simulink model "c00004M_harness"  (R2018a)
settings: Solver=FixedStepAuto  StartTime=0.0  StopTime=300  FixedStep=0.1  RelTol=1e-3
undefined symbols (not defined in the file): A1, hmax, R1, R2, sigbuilder_block, TempThreshold
(part 4 of 14)

== system c00004M_harness/M176/Tank3 ==
  CT3 : Inport
  F3 : Inport  Port=2
  E3 : Inport  Port=3
  MR3 : Inport  Port=4
  T3 : Inport  Port=5
  EB3 : Inport  Port=6
  Control : Subsystem
  Memory : Memory
  TankModel : Subsystem
  LL3 : Outport
  wires:
  TankModel/1(LiquidLevel) -> Memory/1, LL3/1
  Control/2(LiquidOut) -> TankModel/2(LiquidOut)
  Memory/1 -> Control/8(LiquidLevel)
  MR3/1 -> Control/3(ManualReference)
  CT3/1 -> Control/2(StartMaintenance), Control/1(ControlType)
  F3/1 -> Control/4(Fill)
  E3/1 -> Control/5(Empty)
  EB3/1 -> Control/6(EmergencyButton)
  T3/1 -> Control/7(Temperature)
  Control/1(LiquidIn) -> TankModel/1(LiquidIn)

== system c00004M_harness/M177/Tank3 ==
  CT3 : Inport
  F3 : Inport  Port=2
  E3 : Inport  Port=3
  MR3 : Inport  Port=4
  T3 : Inport  Port=5
  EB3 : Inport  Port=6
  Control : Subsystem
  Memory : Memory
  TankModel : Subsystem
  LL3 : Outport
  wires:
  TankModel/1(LiquidLevel) -> Memory/1, LL3/1
  Control/2(LiquidOut) -> TankModel/2(LiquidOut)
  Memory/1 -> Control/8(LiquidLevel)
  MR3/1 -> Control/3(ManualReference)
  CT3/1 -> Control/2(StartMaintenance), Control/1(ControlType)
  F3/1 -> Control/4(Fill)
  E3/1 -> Control/5(Empty)
  EB3/1 -> Control/6(EmergencyButton)
  T3/1 -> Control/7(Temperature)
  Control/1(LiquidIn) -> TankModel/1(LiquidIn)

== system c00004M_harness/M178/Tank3 ==
  CT3 : Inport
  F3 : Inport  Port=2
  E3 : Inport  Port=3
  MR3 : Inport  Port=4
  T3 : Inport  Port=5
  EB3 : Inport  Port=6
  Control : Subsystem
  Memory : Memory
  TankModel : Subsystem
  LL3 : Outport
  wires:
  TankModel/1(LiquidLevel) -> Memory/1, LL3/1
  Control/2(LiquidOut) -> TankModel/2(LiquidOut)
  Memory/1 -> Control/8(LiquidLevel)
  MR3/1 -> Control/3(ManualReference)
  CT3/1 -> Control/2(StartMaintenance), Control/1(ControlType)
  F3/1 -> Control/4(Fill)
  E3/1 -> Control/5(Empty)
  EB3/1 -> Control/6(EmergencyButton)
  T3/1 -> Control/7(Temperature)
  Control/1(LiquidIn) -> TankModel/1(LiquidIn)

== system c00004M_harness/M179/Tank3 ==
  CT3 : Inport
  F3 : Inport  Port=2
  E3 : Inport  Port=3
  MR3 : Inport  Port=4
  T3 : Inport  Port=5
  EB3 : Inport  Port=6
  Control : Subsystem
  Memory : Memory
  TankModel : Subsystem
  LL3 : Outport
  wires:
  TankModel/1(LiquidLevel) -> Memory/1, LL3/1
  Control/2(LiquidOut) -> TankModel/2(LiquidOut)
  Memory/1 -> Control/8(LiquidLevel)
  MR3/1 -> Control/3(ManualReference)
  CT3/1 -> Control/2(StartMaintenance), Control/1(ControlType)
  F3/1 -> Control/4(Fill)
  E3/1 -> Control/5(Empty)
  EB3/1 -> Control/6(EmergencyButton)
  T3/1 -> Control/7(Temperature)
  Control/1(LiquidIn) -> TankModel/1(LiquidIn)

== system c00004M_harness/M180/Tank3 ==
  CT3 : Inport
  F3 : Inport  Port=2
  E3 : Inport  Port=3
  MR3 : Inport  Port=4
  T3 : Inport  Port=5
  EB3 : Inport  Port=6
  Control : Subsystem
  Memory : Memory
  TankModel : Subsystem
  LL3 : Outport
  wires:
  TankModel/1(LiquidLevel) -> Memory/1, LL3/1
  Control/2(LiquidOut) -> TankModel/2(LiquidOut)
  Memory/1 -> Control/8(LiquidLevel)
  MR3/1 -> Control/3(ManualReference)
  CT3/1 -> Control/2(StartMaintenance), Control/1(ControlType)
  F3/1 -> Control/4(Fill)
  E3/1 -> Control/5(Empty)
  EB3/1 -> Control/6(EmergencyButton)
  T3/1 -> Control/7(Temperature)
  Control/1(LiquidIn) -> TankModel/1(LiquidIn)

== system c00004M_harness/M181/Tank3 ==
  CT3 : Inport
  F3 : Inport  Port=2
  E3 : Inport  Port=3
  MR3 : Inport  Port=4
  T3 : Inport  Port=5
  EB3 : Inport  Port=6
  Control : Subsystem
  Memory : Memory
  TankModel : Subsystem
  LL3 : Outport
  wires:
  TankModel/1(LiquidLevel) -> Memory/1, LL3/1
  Control/2(LiquidOut) -> TankModel/2(LiquidOut)
  Memory/1 -> Control/8(LiquidLevel)
  MR3/1 -> Control/3(ManualReference)
  CT3/1 -> Control/2(StartMaintenance), Control/1(ControlType)
  F3/1 -> Control/4(Fill)
  E3/1 -> Control/5(Empty)
  EB3/1 -> Control/6(EmergencyButton)
  T3/1 -> Control/7(Temperature)
  Control/1(LiquidIn) -> TankModel/1(LiquidIn)

== system c00004M_harness/M182/Tank3 ==
  CT3 : Inport
  F3 : Inport  Port=2
  E3 : Inport  Port=3
  MR3 : Inport  Port=4
  T3 : Inport  Port=5
  EB3 : Inport  Port=6
  Control : Subsystem
  Memory : Memory
  TankModel : Subsystem
  LL3 : Outport
  wires:
  TankModel/1(LiquidLevel) -> Memory/1, LL3/1
  Control/2(LiquidOut) -> TankModel/2(LiquidOut)
  Memory/1 -> Control/8(LiquidLevel)
  MR3/1 -> Control/3(ManualReference)
  CT3/1 -> Control/2(StartMaintenance), Control/1(ControlType)
  F3/1 -> Control/4(Fill)
  E3/1 -> Control/5(Empty)
  EB3/1 -> Control/6(EmergencyButton)
  T3/1 -> Control/7(Temperature)
  Control/1(LiquidIn) -> TankModel/1(LiquidIn)

== system c00004M_harness/M183/Tank3 ==
  CT3 : Inport
  F3 : Inport  Port=2
  E3 : Inport  Port=3
  MR3 : Inport  Port=4
  T3 : Inport  Port=5
  EB3 : Inport  Port=6
  Control : Subsystem
  Memory : Memory
  TankModel : Subsystem
  LL3 : Outport
  wires:
  TankModel/1(LiquidLevel) -> Memory/1, LL3/1
  Control/2(LiquidOut) -> TankModel/2(LiquidOut)
  Memory/1 -> Control/8(LiquidLevel)
  MR3/1 -> Control/3(ManualReference)
  CT3/1 -> Control/2(StartMaintenance), Control/1(ControlType)
  F3/1 -> Control/4(Fill)
  E3/1 -> Control/5(Empty)
  EB3/1 -> Control/6(EmergencyButton)
  T3/1 -> Control/7(Temperature)
  Control/1(LiquidIn) -> TankModel/1(LiquidIn)

== system c00004M_harness/M184/Tank3 ==
  CT3 : Inport
  F3 : Inport  Port=2
  E3 : Inport  Port=3
  MR3 : Inport  Port=4
  T3 : Inport  Port=5
  EB3 : Inport  Port=6
  Control : Subsystem
  Memory : Memory
  TankModel : Subsystem
  LL3 : Outport
  wires:
  TankModel/1(LiquidLevel) -> Memory/1, LL3/1
  Control/2(LiquidOut) -> TankModel/2(LiquidOut)
  Memory/1 -> Control/8(LiquidLevel)
  MR3/1 -> Control/3(ManualReference)
  CT3/1 -> Control/2(StartMaintenance), Control/1(ControlType)
  F3/1 -> Control/4(Fill)
  E3/1 -> Control/5(Empty)
  EB3/1 -> Control/6(EmergencyButton)
  T3/1 -> Control/7(Temperature)
  Control/1(LiquidIn) -> TankModel/1(LiquidIn)

== system c00004M_harness/M185/Tank3 ==
  CT3 : Inport
  F3 : Inport  Port=2
  E3 : Inport  Port=3
  MR3 : Inport  Port=4
  T3 : Inport  Port=5
  EB3 : Inport  Port=6
  Control : Subsystem
  Memory : Memory
  TankModel : Subsystem
  LL3 : Outport
  wires:
  TankModel/1(LiquidLevel) -> Memory/1, LL3/1
  Control/2(LiquidOut) -> TankModel/2(LiquidOut)
  Memory/1 -> Control/8(LiquidLevel)
  MR3/1 -> Control/3(ManualReference)
  CT3/1 -> Control/2(StartMaintenance), Control/1(ControlType)
  F3/1 -> Control/4(Fill)
  E3/1 -> Control/5(Empty)
  EB3/1 -> Control/6(EmergencyButton)
  T3/1 -> Control/7(Temperature)
  Control/1(LiquidIn) -> TankModel/1(LiquidIn)

== system c00004M_harness/M186/Tank3 ==
  CT3 : Inport
  F3 : Inport  Port=2
  E3 : Inport  Port=3
  MR3 : Inport  Port=4
  T3 : Inport  Port=5
  EB3 : Inport  Port=6
  Control : Subsystem
  Memory : Memory
  TankModel : Subsystem
  LL3 : Outport
  wires:
  TankModel/1(LiquidLevel) -> Memory/1, LL3/1
  Control/2(LiquidOut) -> TankModel/2(LiquidOut)
  Memory/1 -> Control/8(LiquidLevel)
  MR3/1 -> Control/3(ManualReference)
  CT3/1 -> Control/2(StartMaintenance), Control/1(ControlType)
  F3/1 -> Control/4(Fill)
  E3/1 -> Control/5(Empty)
  EB3/1 -> Control/6(EmergencyButton)
  T3/1 -> Control/7(Temperature)
  Control/1(LiquidIn) -> TankModel/1(LiquidIn)

== system c00004M_harness/M187/Tank3 ==
  CT3 : Inport
  F3 : Inport  Port=2
  E3 : Inport  Port=3
  MR3 : Inport  Port=4
  T3 : Inport  Port=5
  EB3 : Inport  Port=6
  Control : Subsystem
  Memory : Memory
  TankModel : Subsystem
  LL3 : Outport
  wires:
  TankModel/1(LiquidLevel) -> Memory/1, LL3/1
  Control/2(LiquidOut) -> TankModel/2(LiquidOut)
  Memory/1 -> Control/8(LiquidLevel)
  MR3/1 -> Control/3(ManualReference)
  CT3/1 -> Control/2(StartMaintenance), Control/1(ControlType)
  F3/1 -> Control/4(Fill)
  E3/1 -> Control/5(Empty)
  EB3/1 -> Control/6(EmergencyButton)
  T3/1 -> Control/7(Temperature)
  Control/1(LiquidIn) -> TankModel/1(LiquidIn)

== system c00004M_harness/M188/Tank3 ==
  CT3 : Inport
  F3 : Inport  Port=2
  E3 : Inport  Port=3
  MR3 : Inport  Port=4
  T3 : Inport  Port=5
  EB3 : Inport  Port=6
  Control : Subsystem
  Memory : Memory
  TankModel : Subsystem
  LL3 : Outport
  wires:
  TankModel/1(LiquidLevel) -> Memory/1, LL3/1
  Control/2(LiquidOut) -> TankModel/2(LiquidOut)
  Memory/1 -> Control/8(LiquidLevel)
  MR3/1 -> Control/3(ManualReference)
  CT3/1 -> Control/2(StartMaintenance), Control/1(ControlType)
  F3/1 -> Control/4(Fill)
  E3/1 -> Control/5(Empty)
  EB3/1 -> Control/6(EmergencyButton)
  T3/1 -> Control/7(Temperature)
  Control/1(LiquidIn) -> TankModel/1(LiquidIn)

== system c00004M_harness/M189/Tank3 ==
  CT3 : Inport
  F3 : Inport  Port=2
  E3 : Inport  Port=3
  MR3 : Inport  Port=4
  T3 : Inport  Port=5
  EB3 : Inport  Port=6
  Control : Subsystem
  Memory : Memory
  TankModel : Subsystem
  LL3 : Outport
  wires:
  TankModel/1(LiquidLevel) -> Memory/1, LL3/1
  Control/2(LiquidOut) -> TankModel/2(LiquidOut)
  Memory/1 -> Control/8(LiquidLevel)
  MR3/1 -> Control/3(ManualReference)
  CT3/1 -> Control/2(StartMaintenance), Control/1(ControlType)
  F3/1 -> Control/4(Fill)
  E3/1 -> Control/5(Empty)
  EB3/1 -> Control/6(EmergencyButton)
  T3/1 -> Control/7(Temperature)
  Control/1(LiquidIn) -> TankModel/1(LiquidIn)

== system c00004M_harness/M190/Tank3 ==
  CT3 : Inport
  F3 : Inport  Port=2
  E3 : Inport  Port=3
  MR3 : Inport  Port=4
  T3 : Inport  Port=5
  EB3 : Inport  Port=6
  Control : Subsystem
  Memory : Memory
  TankModel : Subsystem
  LL3 : Outport
  wires:
  TankModel/1(LiquidLevel) -> Memory/1, LL3/1
  Control/2(LiquidOut) -> TankModel/2(LiquidOut)
  Memory/1 -> Control/8(LiquidLevel)
  MR3/1 -> Control/3(ManualReference)
  CT3/1 -> Control/2(StartMaintenance), Control/1(ControlType)
  F3/1 -> Control/4(Fill)
  E3/1 -> Control/5(Empty)
  EB3/1 -> Control/6(EmergencyButton)
  T3/1 -> Control/7(Temperature)
  Control/1(LiquidIn) -> TankModel/1(LiquidIn)

== system c00004M_harness/M191/Tank3 ==
  CT3 : Inport
  F3 : Inport  Port=2
  E3 : Inport  Port=3
  MR3 : Inport  Port=4
  T3 : Inport  Port=5
  EB3 : Inport  Port=6
  Control : Subsystem
  Memory : Memory
  TankModel : Subsystem
  LL3 : Outport
  wires:
  TankModel/1(LiquidLevel) -> Memory/1, LL3/1
  Control/2(LiquidOut) -> TankModel/2(LiquidOut)
  Memory/1 -> Control/8(LiquidLevel)
  MR3/1 -> Control/3(ManualReference)
  CT3/1 -> Control/2(StartMaintenance), Control/1(ControlType)
  F3/1 -> Control/4(Fill)
  E3/1 -> Control/5(Empty)
  EB3/1 -> Control/6(EmergencyButton)
  T3/1 -> Control/7(Temperature)
  Control/1(LiquidIn) -> TankModel/1(LiquidIn)

== system c00004M_harness/M192/Tank3 ==
  CT3 : Inport
  F3 : Inport  Port=2
  E3 : Inport  Port=3
  MR3 : Inport  Port=4
  T3 : Inport  Port=5
  EB3 : Inport  Port=6
  Control : Subsystem
  Memory : Memory
  TankModel : Subsystem
  LL3 : Outport
  wires:
  TankModel/1(LiquidLevel) -> Memory/1, LL3/1
  Control/2(LiquidOut) -> TankModel/2(LiquidOut)
  Memory/1 -> Control/8(LiquidLevel)
  MR3/1 -> Control/3(ManualReference)
  CT3/1 -> Control/2(StartMaintenance), Control/1(ControlType)
  F3/1 -> Control/4(Fill)
  E3/1 -> Control/5(Empty)
  EB3/1 -> Control/6(EmergencyButton)
  T3/1 -> Control/7(Temperature)
  Control/1(LiquidIn) -> TankModel/1(LiquidIn)

== system c00004M_harness/M193/Tank3 ==
  CT3 : Inport
  F3 : Inport  Port=2
  E3 : Inport  Port=3
  MR3 : Inport  Port=4
  T3 : Inport  Port=5
  EB3 : Inport  Port=6
  Control : Subsystem
  Memory : Memory
  TankModel : Subsystem
  LL3 : Outport
  wires:
  TankModel/1(LiquidLevel) -> Memory/1, LL3/1
  Control/2(LiquidOut) -> TankModel/2(LiquidOut)
  Memory/1 -> Control/8(LiquidLevel)
  MR3/1 -> Control/3(ManualReference)
  CT3/1 -> Control/2(StartMaintenance), Control/1(ControlType)
  F3/1 -> Control/4(Fill)
  E3/1 -> Control/5(Empty)
  EB3/1 -> Control/6(EmergencyButton)
  T3/1 -> Control/7(Temperature)
  Control/1(LiquidIn) -> TankModel/1(LiquidIn)

== system c00004M_harness/M194/Tank3 ==
  CT3 : Inport
  F3 : Inport  Port=2
  E3 : Inport  Port=3
  MR3 : Inport  Port=4
  T3 : Inport  Port=5
  EB3 : Inport  Port=6
  Control : Subsystem
  Memory : Memory
  TankModel : Subsystem
  LL3 : Outport
  wires:
  TankModel/1(LiquidLevel) -> Memory/1, LL3/1
  Control/2(LiquidOut) -> TankModel/2(LiquidOut)
  Memory/1 -> Control/8(LiquidLevel)
  MR3/1 -> Control/3(ManualReference)
  CT3/1 -> Control/2(StartMaintenance), Control/1(ControlType)
  F3/1 -> Control/4(Fill)
  E3/1 -> Control/5(Empty)
  EB3/1 -> Control/6(EmergencyButton)
  T3/1 -> Control/7(Temperature)
  Control/1(LiquidIn) -> TankModel/1(LiquidIn)

== system c00004M_harness/M195/Tank3 ==
  CT3 : Inport
  F3 : Inport  Port=2
  E3 : Inport  Port=3
  MR3 : Inport  Port=4
  T3 : Inport  Port=5
  EB3 : Inport  Port=6
  Control : Subsystem
  Memory : Memory
  TankModel : Subsystem
  LL3 : Outport
  wires:
  TankModel/1(LiquidLevel) -> Memory/1, LL3/1
  Control/2(LiquidOut) -> TankModel/2(LiquidOut)
  Memory/1 -> Control/8(LiquidLevel)
  MR3/1 -> Control/3(ManualReference)
  CT3/1 -> Control/2(StartMaintenance), Control/1(ControlType)
  F3/1 -> Control/4(Fill)
  E3/1 -> Control/5(Empty)
  EB3/1 -> Control/6(EmergencyButton)
  T3/1 -> Control/7(Temperature)
  Control/1(LiquidIn) -> TankModel/1(LiquidIn)

== system c00004M_harness/M196/Tank3 ==
  CT3 : Inport
  F3 : Inport  Port=2
  E3 : Inport  Port=3
  MR3 : Inport  Port=4
  T3 : Inport  Port=5
  EB3 : Inport  Port=6
  Control : Subsystem
  Memory : Memory
  TankModel : Subsystem
  LL3 : Outport
  wires:
  TankModel/1(LiquidLevel) -> Memory/1, LL3/1
  Control/2(LiquidOut) -> TankModel/2(LiquidOut)
  Memory/1 -> Control/8(LiquidLevel)
  MR3/1 -> Control/3(ManualReference)
  CT3/1 -> Control/2(StartMaintenance), Control/1(ControlType)
  F3/1 -> Control/4(Fill)
  E3/1 -> Control/5(Empty)
  EB3/1 -> Control/6(EmergencyButton)
  T3/1 -> Control/7(Temperature)
  Control/1(LiquidIn) -> TankModel/1(LiquidIn)

== system c00004M_harness/M197/Tank3 ==
  CT3 : Inport
  F3 : Inport  Port=2
  E3 : Inport  Port=3
  MR3 : Inport  Port=4
  T3 : Inport  Port=5
  EB3 : Inport  Port=6
  Control : Subsystem
  Memory : Memory
  TankModel : Subsystem
  LL3 : Outport
  wires:
  TankModel/1(LiquidLevel) -> Memory/1, LL3/1
  Control/2(LiquidOut) -> TankModel/2(LiquidOut)
  Memory/1 -> Control/8(LiquidLevel)
  MR3/1 -> Control/3(ManualReference)
  CT3/1 -> Control/2(StartMaintenance), Control/1(ControlType)
  F3/1 -> Control/4(Fill)
  E3/1 -> Control/5(Empty)
  EB3/1 -> Control/6(EmergencyButton)
  T3/1 -> Control/7(Temperature)
  Control/1(LiquidIn) -> TankModel/1(LiquidIn)

== system c00004M_harness/M198/Tank3 ==
  CT3 : Inport
  F3 : Inport  Port=2
  E3 : Inport  Port=3
  MR3 : Inport  Port=4
  T3 : Inport  Port=5
  EB3 : Inport  Port=6
  Control : Subsystem
  Memory : Memory
  TankModel : Subsystem
  LL3 : Outport
  wires:
  TankModel/1(LiquidLevel) -> Memory/1, LL3/1
  Control/2(LiquidOut) -> TankModel/2(LiquidOut)
  Memory/1 -> Control/8(LiquidLevel)
  MR3/1 -> Control/3(ManualReference)
  CT3/1 -> Control/2(StartMaintenance), Control/1(ControlType)
  F3/1 -> Control/4(Fill)
  E3/1 -> Control/5(Empty)
  EB3/1 -> Control/6(EmergencyButton)
  T3/1 -> Control/7(Temperature)
  Control/1(LiquidIn) -> TankModel/1(LiquidIn)

== system c00004M_harness/M199/Tank3 ==
  CT3 : Inport
  F3 : Inport  Port=2
  E3 : Inport  Port=3
  MR3 : Inport  Port=4
  T3 : Inport  Port=5
  EB3 : Inport  Port=6
  Control : Subsystem
  Memory : Memory
  TankModel : Subsystem
  LL3 : Outport
  wires:
  TankModel/1(LiquidLevel) -> Memory/1, LL3/1
  Control/2(LiquidOut) -> TankModel/2(LiquidOut)
  Memory/1 -> Control/8(LiquidLevel)
  MR3/1 -> Control/3(ManualReference)
  CT3/1 -> Control/2(StartMaintenance), Control/1(ControlType)
  F3/1 -> Control/4(Fill)
  E3/1 -> Control/5(Empty)
  EB3/1 -> Control/6(EmergencyButton)
  T3/1 -> Control/7(Temperature)
  Control/1(LiquidIn) -> TankModel/1(LiquidIn)

== system c00004M_harness/M200/Tank3 ==
  CT3 : Inport
  F3 : Inport  Port=2
  E3 : Inport  Port=3
  MR3 : Inport  Port=4
  T3 : Inport  Port=5
  EB3 : Inport  Port=6
  Control : Subsystem
  Memory : Memory
  TankModel : Subsystem
  LL3 : Outport
  wires:
  TankModel/1(LiquidLevel) -> Memory/1, LL3/1
  Control/2(LiquidOut) -> TankModel/2(LiquidOut)
  Memory/1 -> Control/8(LiquidLevel)
  MR3/1 -> Control/3(ManualReference)
  CT3/1 -> Control/2(StartMaintenance), Control/1(ControlType)
  F3/1 -> Control/4(Fill)
  E3/1 -> Control/5(Empty)
  EB3/1 -> Control/6(EmergencyButton)
  T3/1 -> Control/7(Temperature)
  Control/1(LiquidIn) -> TankModel/1(LiquidIn)

== system c00004M_harness/M201/Tank3 ==
  CT3 : Inport
  F3 : Inport  Port=2
  E3 : Inport  Port=3
  MR3 : Inport  Port=4
  T3 : Inport  Port=5
  EB3 : Inport  Port=6
  Control : Subsystem
  Memory : Memory
  TankModel : Subsystem
  LL3 : Outport
  wires:
  TankModel/1(LiquidLevel) -> Memory/1, LL3/1
  Control/2(LiquidOut) -> TankModel/2(LiquidOut)
  Memory/1 -> Control/8(LiquidLevel)
  MR3/1 -> Control/3(ManualReference)
  CT3/1 -> Control/2(StartMaintenance), Control/1(ControlType)
  F3/1 -> Control/4(Fill)
  E3/1 -> Control/5(Empty)
  EB3/1 -> Control/6(EmergencyButton)
  T3/1 -> Control/7(Temperature)
  Control/1(LiquidIn) -> TankModel/1(LiquidIn)

== system c00004M_harness/M202/Tank3 ==
  CT3 : Inport
  F3 : Inport  Port=2
  E3 : Inport  Port=3
  MR3 : Inport  Port=4
  T3 : Inport  Port=5
  EB3 : Inport  Port=6
  Control : Subsystem
  Memory : Memory
  TankModel : Subsystem
  LL3 : Outport
  wires:
  TankModel/1(LiquidLevel) -> Memory/1, LL3/1
  Control/2(LiquidOut) -> TankModel/2(LiquidOut)
  Memory/1 -> Control/8(LiquidLevel)
  MR3/1 -> Control/3(ManualReference)
  CT3/1 -> Control/2(StartMaintenance), Control/1(ControlType)
  F3/1 -> Control/4(Fill)
  E3/1 -> Control/5(Empty)
  EB3/1 -> Control/6(EmergencyButton)
  T3/1 -> Control/7(Temperature)
  Control/1(LiquidIn) -> TankModel/1(LiquidIn)

== system c00004M_harness/M203/Tank3 ==
  CT3 : Inport
  F3 : Inport  Port=2
  E3 : Inport  Port=3
  MR3 : Inport  Port=4
  T3 : Inport  Port=5
  EB3 : Inport  Port=6
  Control : Subsystem
  Memory : Memory
  TankModel : Subsystem
  LL3 : Outport
  wires:
  TankModel/1(LiquidLevel) -> Memory/1, LL3/1
  Control/2(LiquidOut) -> TankModel/2(LiquidOut)
  Memory/1 -> Control/8(LiquidLevel)
  MR3/1 -> Control/3(ManualReference)
  CT3/1 -> Control/2(StartMaintenance), Control/1(ControlType)
  F3/1 -> Control/4(Fill)
  E3/1 -> Control/5(Empty)
  EB3/1 -> Control/6(EmergencyButton)
  T3/1 -> Control/7(Temperature)
  Control/1(LiquidIn) -> TankModel/1(LiquidIn)

== system c00004M_harness/M204/Tank3 ==
  CT3 : Inport
  F3 : Inport  Port=2
  E3 : Inport  Port=3
  MR3 : Inport  Port=4
  T3 : Inport  Port=5
  EB3 : Inport  Port=6
  Control : Subsystem
  Memory : Memory
  TankModel : Subsystem
  LL3 : Outport
  wires:
  TankModel/1(LiquidLevel) -> Memory/1, LL3/1
  Control/2(LiquidOut) -> TankModel/2(LiquidOut)
  Memory/1 -> Control/8(LiquidLevel)
  MR3/1 -> Control/3(ManualReference)
  CT3/1 -> Control/2(StartMaintenance), Control/1(ControlType)
  F3/1 -> Control/4(Fill)
  E3/1 -> Control/5(Empty)
  EB3/1 -> Control/6(EmergencyButton)
  T3/1 -> Control/7(Temperature)
  Control/1(LiquidIn) -> TankModel/1(LiquidIn)

== system c00004M_harness/M205/Tank3 ==
  CT3 : Inport
  F3 : Inport  Port=2
  E3 : Inport  Port=3
  MR3 : Inport  Port=4
  T3 : Inport  Port=5
  EB3 : Inport  Port=6
  Control : Subsystem
  Memory : Memory
  TankModel : Subsystem
  LL3 : Outport
  wires:
  TankModel/1(LiquidLevel) -> Memory/1, LL3/1
  Control/2(LiquidOut) -> TankModel/2(LiquidOut)
  Memory/1 -> Control/8(LiquidLevel)
  MR3/1 -> Control/3(ManualReference)
  CT3/1 -> Control/2(StartMaintenance), Control/1(ControlType)
  F3/1 -> Control/4(Fill)
  E3/1 -> Control/5(Empty)
  EB3/1 -> Control/6(EmergencyButton)
  T3/1 -> Control/7(Temperature)
  Control/1(LiquidIn) -> TankModel/1(LiquidIn)

== system c00004M_harness/M206/Tank3 ==
  CT3 : Inport
  F3 : Inport  Port=2
  E3 : Inport  Port=3
  MR3 : Inport  Port=4
  T3 : Inport  Port=5
  EB3 : Inport  Port=6
  Control : Subsystem
  Memory : Memory
  TankModel : Subsystem
  LL3 : Outport
  wires:
  TankModel/1(LiquidLevel) -> Memory/1, LL3/1
  Control/2(LiquidOut) -> TankModel/2(LiquidOut)
  Memory/1 -> Control/8(LiquidLevel)
  MR3/1 -> Control/3(ManualReference)
  CT3/1 -> Control/2(StartMaintenance), Control/1(ControlType)
  F3/1 -> Control/4(Fill)
  E3/1 -> Control/5(Empty)
  EB3/1 -> Control/6(EmergencyButton)
  T3/1 -> Control/7(Temperature)
  Control/1(LiquidIn) -> TankModel/1(LiquidIn)

== system c00004M_harness/M207/Tank3 ==
  CT3 : Inport
  F3 : Inport  Port=2
  E3 : Inport  Port=3
  MR3 : Inport  Port=4
  T3 : Inport  Port=5
  EB3 : Inport  Port=6
  Control : Subsystem
  Memory : Memory
  TankModel : Subsystem
  LL3 : Outport
  wires:
  TankModel/1(LiquidLevel) -> Memory/1, LL3/1
  Control/2(LiquidOut) -> TankModel/2(LiquidOut)
  Memory/1 -> Control/8(LiquidLevel)
  MR3/1 -> Control/3(ManualReference)
  CT3/1 -> Control/2(StartMaintenance), Control/1(ControlType)
  F3/1 -> Control/4(Fill)
  E3/1 -> Control/5(Empty)
  EB3/1 -> Control/6(EmergencyButton)
  T3/1 -> Control/7(Temperature)
  Control/1(LiquidIn) -> TankModel/1(LiquidIn)

== system c00004M_harness/M208/Tank3 ==
  CT3 : Inport
  F3 : Inport  Port=2
  E3 : Inport  Port=3
  MR3 : Inport  Port=4
  T3 : Inport  Port=5
  EB3 : Inport  Port=6
  Control : Subsystem
  Memory : Memory
  TankModel : Subsystem
  LL3 : Outport
  wires:
  TankModel/1(LiquidLevel) -> Memory/1, LL3/1
  Control/2(LiquidOut) -> TankModel/2(LiquidOut)
  Memory/1 -> Control/8(LiquidLevel)
  MR3/1 -> Control/3(ManualReference)
  CT3/1 -> Control/2(StartMaintenance), Control/1(ControlType)
  F3/1 -> Control/4(Fill)
  E3/1 -> Control/5(Empty)
  EB3/1 -> Control/6(EmergencyButton)
  T3/1 -> Control/7(Temperature)
  Control/1(LiquidIn) -> TankModel/1(LiquidIn)

== system c00004M_harness/M209/Tank3 ==
  CT3 : Inport
  F3 : Inport  Port=2
  E3 : Inport  Port=3
  MR3 : Inport  Port=4
  T3 : Inport  Port=5
  EB3 : Inport  Port=6
  Control : Subsystem
  Memory : Memory
  TankModel : Subsystem
  LL3 : Outport
  wires:
  TankModel/1(LiquidLevel) -> Memory/1, LL3/1
  Control/2(LiquidOut) -> TankModel/2(LiquidOut)
  Memory/1 -> Control/8(LiquidLevel)
  MR3/1 -> Control/3(ManualReference)
  CT3/1 -> Control/2(StartMaintenance), Control/1(ControlType)
  F3/1 -> Control/4(Fill)
  E3/1 -> Control/5(Empty)
  EB3/1 -> Control/6(EmergencyButton)
  T3/1 -> Control/7(Temperature)
  Control/1(LiquidIn) -> TankModel/1(LiquidIn)

== system c00004M_harness/M210/Tank3 ==
  CT3 : Inport
  F3 : Inport  Port=2
  E3 : Inport  Port=3
  MR3 : Inport  Port=4
  T3 : Inport  Port=5
  EB3 : Inport  Port=6
  Control : Subsystem
  Memory : Memory
  TankModel : Subsystem
  LL3 : Outport
  wires:
  TankModel/1(LiquidLevel) -> Memory/1, LL3/1
  Control/2(LiquidOut) -> TankModel/2(LiquidOut)
  Memory/1 -> Control/8(LiquidLevel)
  MR3/1 -> Control/3(ManualReference)
  CT3/1 -> Control/2(StartMaintenance), Control/1(ControlType)
  F3/1 -> Control/4(Fill)
  E3/1 -> Control/5(Empty)
  EB3/1 -> Control/6(EmergencyButton)
  T3/1 -> Control/7(Temperature)
  Control/1(LiquidIn) -> TankModel/1(LiquidIn)

== system c00004M_harness/M211/Tank3 ==
  CT3 : Inport
  F3 : Inport  Port=2
  E3 : Inport  Port=3
  MR3 : Inport  Port=4
  T3 : Inport  Port=5
  EB3 : Inport  Port=6
  Control : Subsystem
  Memory : Memory
  TankModel : Subsystem
  LL3 : Outport
  wires:
  TankModel/1(LiquidLevel) -> Memory/1, LL3/1
  Control/2(LiquidOut) -> TankModel/2(LiquidOut)
  Memory/1 -> Control/8(LiquidLevel)
  MR3/1 -> Control/3(ManualReference)
  CT3/1 -> Control/2(StartMaintenance), Control/1(ControlType)
  F3/1 -> Control/4(Fill)
  E3/1 -> Control/5(Empty)
  EB3/1 -> Control/6(EmergencyButton)
  T3/1 -> Control/7(Temperature)
  Control/1(LiquidIn) -> TankModel/1(LiquidIn)

== system c00004M_harness/M212/Tank3 ==
  CT3 : Inport
  F3 : Inport  Port=2
  E3 : Inport  Port=3
  MR3 : Inport  Port=4
  T3 : Inport  Port=5
  EB3 : Inport  Port=6
  Control : Subsystem
  Memory : Memory
  TankModel : Subsystem
  LL3 : Outport
  wires:
  TankModel/1(LiquidLevel) -> Memory/1, LL3/1
  Control/2(LiquidOut) -> TankModel/2(LiquidOut)
  Memory/1 -> Control/8(LiquidLevel)
  MR3/1 -> Control/3(ManualReference)
  CT3/1 -> Control/2(StartMaintenance), Control/1(ControlType)
  F3/1 -> Control/4(Fill)
  E3/1 -> Control/5(Empty)
  EB3/1 -> Control/6(EmergencyButton)
  T3/1 -> Control/7(Temperature)
  Control/1(LiquidIn) -> TankModel/1(LiquidIn)

== system c00004M_harness/M213/Tank3 ==
  CT3 : Inport
  F3 : Inport  Port=2
  E3 : Inport  Port=3
  MR3 : Inport  Port=4
  T3 : Inport  Port=5
  EB3 : Inport  Port=6
  Control : Subsystem
  Memory : Memory
  TankModel : Subsystem
  LL3 : Outport
  wires:
  TankModel/1(LiquidLevel) -> Memory/1, LL3/1
  Control/2(LiquidOut) -> TankModel/2(LiquidOut)
  Memory/1 -> Control/8(LiquidLevel)
  MR3/1 -> Control/3(ManualReference)
  CT3/1 -> Control/2(StartMaintenance), Control/1(ControlType)
  F3/1 -> Control/4(Fill)
  E3/1 -> Control/5(Empty)
  EB3/1 -> Control/6(EmergencyButton)
  T3/1 -> Control/7(Temperature)
  Control/1(LiquidIn) -> TankModel/1(LiquidIn)

== system c00004M_harness/M214/Tank3 ==
  CT3 : Inport
  F3 : Inport  Port=2
  E3 : Inport  Port=3
  MR3 : Inport  Port=4
  T3 : Inport  Port=5
  EB3 : Inport  Port=6
  Control : Subsystem
  Memory : Memory
  TankModel : Subsystem
  LL3 : Outport
  wires:
  TankModel/1(LiquidLevel) -> Memory/1, LL3/1
  Control/2(LiquidOut) -> TankModel/2(LiquidOut)
  Memory/1 -> Control/8(LiquidLevel)
  MR3/1 -> Control/3(ManualReference)
  CT3/1 -> Control/2(StartMaintenance), Control/1(ControlType)
  F3/1 -> Control/4(Fill)
  E3/1 -> Control/5(Empty)
  EB3/1 -> Control/6(EmergencyButton)
  T3/1 -> Control/7(Temperature)
  Control/1(LiquidIn) -> TankModel/1(LiquidIn)

== system c00004M_harness/M215/Tank3 ==
  CT3 : Inport
  F3 : Inport  Port=2
  E3 : Inport  Port=3
  MR3 : Inport  Port=4
  T3 : Inport  Port=5
  EB3 : Inport  Port=6
  Control : Subsystem
  Memory : Memory
  TankModel : Subsystem
  LL3 : Outport
  wires:
  TankModel/1(LiquidLevel) -> Memory/1, LL3/1
  Control/2(LiquidOut) -> TankModel/2(LiquidOut)
  Memory/1 -> Control/8(LiquidLevel)
  MR3/1 -> Control/3(ManualReference)
  CT3/1 -> Control/2(StartMaintenance), Control/1(ControlType)
  F3/1 -> Control/4(Fill)
  E3/1 -> Control/5(Empty)
  EB3/1 -> Control/6(EmergencyButton)
  T3/1 -> Control/7(Temperature)
  Control/1(LiquidIn) -> TankModel/1(LiquidIn)

== system c00004M_harness/M216/Tank3 ==
  CT3 : Inport
  F3 : Inport  Port=2
  E3 : Inport  Port=3
  MR3 : Inport  Port=4
  T3 : Inport  Port=5
  EB3 : Inport  Port=6
  Control : Subsystem
  Memory : Memory
  TankModel : Subsystem
  LL3 : Outport
  wires:
  TankModel/1(LiquidLevel) -> Memory/1, LL3/1
  Control/2(LiquidOut) -> TankModel/2(LiquidOut)
  Memory/1 -> Control/8(LiquidLevel)
  MR3/1 -> Control/3(ManualReference)
  CT3/1 -> Control/2(StartMaintenance), Control/1(ControlType)
  F3/1 -> Control/4(Fill)
  E3/1 -> Control/5(Empty)
  EB3/1 -> Control/6(EmergencyButton)
  T3/1 -> Control/7(Temperature)
  Control/1(LiquidIn) -> TankModel/1(LiquidIn)

== system c00004M_harness/M217/Tank3 ==
  CT3 : Inport
  F3 : Inport  Port=2
  E3 : Inport  Port=3
  MR3 : Inport  Port=4
  T3 : Inport  Port=5
  EB3 : Inport  Port=6
  Control : Subsystem
  Memory : Memory
  TankModel : Subsystem
  LL3 : Outport
  wires:
  TankModel/1(LiquidLevel) -> Memory/1, LL3/1
  Control/2(LiquidOut) -> TankModel/2(LiquidOut)
  Memory/1 -> Control/8(LiquidLevel)
  MR3/1 -> Control/3(ManualReference)
  CT3/1 -> Control/2(StartMaintenance), Control/1(ControlType)
  F3/1 -> Control/4(Fill)
  E3/1 -> Control/5(Empty)
  EB3/1 -> Control/6(EmergencyButton)
  T3/1 -> Control/7(Temperature)
  Control/1(LiquidIn) -> TankModel/1(LiquidIn)

== system c00004M_harness/M218/Tank3 ==
  CT3 : Inport
  F3 : Inport  Port=2
  E3 : Inport  Port=3
  MR3 : Inport  Port=4
  T3 : Inport  Port=5
  EB3 : Inport  Port=6
  Control : Subsystem
  Memory : Memory
  TankModel : Subsystem
  LL3 : Outport
  wires:
  TankModel/1(LiquidLevel) -> Memory/1, LL3/1
  Control/2(LiquidOut) -> TankModel/2(LiquidOut)
  Memory/1 -> Control/8(LiquidLevel)
  MR3/1 -> Control/3(ManualReference)
  CT3/1 -> Control/2(StartMaintenance), Control/1(ControlType)
  F3/1 -> Control/4(Fill)
  E3/1 -> Control/5(Empty)
  EB3/1 -> Control/6(EmergencyButton)
  T3/1 -> Control/7(Temperature)
  Control/1(LiquidIn) -> TankModel/1(LiquidIn)

== system c00004M_harness/M219/Tank3 ==
  CT3 : Inport
  F3 : Inport  Port=2
  E3 : Inport  Port=3
  MR3 : Inport  Port=4
  T3 : Inport  Port=5
  EB3 : Inport  Port=6
  Control : Subsystem
  Memory : Memory
  TankModel : Subsystem
  LL3 : Outport
  wires:
  TankModel/1(LiquidLevel) -> Memory/1, LL3/1
  Control/2(LiquidOut) -> TankModel/2(LiquidOut)
  Memory/1 -> Control/8(LiquidLevel)
  MR3/1 -> Control/3(ManualReference)
  CT3/1 -> Control/2(StartMaintenance), Control/1(ControlType)
  F3/1 -> Control/4(Fill)
  E3/1 -> Control/5(Empty)
  EB3/1 -> Control/6(EmergencyButton)
  T3/1 -> Control/7(Temperature)
  Control/1(LiquidIn) -> TankModel/1(LiquidIn)

== system c00004M_harness/M220/Tank3 ==
  CT3 : Inport
  F3 : Inport  Port=2
  E3 : Inport  Port=3
  MR3 : Inport  Port=4
  T3 : Inport  Port=5
  EB3 : Inport  Port=6
  Control : Subsystem
  Memory : Memory
  TankModel : Subsystem
  LL3 : Outport
  wires:
  TankModel/1(LiquidLevel) -> Memory/1, LL3/1
  Control/2(LiquidOut) -> TankModel/2(LiquidOut)
  Memory/1 -> Control/8(LiquidLevel)
  MR3/1 -> Control/3(ManualReference)
  CT3/1 -> Control/2(StartMaintenance), Control/1(ControlType)
  F3/1 -> Control/4(Fill)
  E3/1 -> Control/5(Empty)
  EB3/1 -> Control/6(EmergencyButton)
  T3/1 -> Control/7(Temperature)
  Control/1(LiquidIn) -> TankModel/1(LiquidIn)

== system c00004M_harness/M221/Tank3 ==
  CT3 : Inport
  F3 : Inport  Port=2
  E3 : Inport  Port=3
  MR3 : Inport  Port=4
  T3 : Inport  Port=5
  EB3 : Inport  Port=6
  Control : Subsystem
  Memory : Memory
  TankModel : Subsystem
  LL3 : Outport
  wires:
  TankModel/1(LiquidLevel) -> Memory/1, LL3/1
  Control/2(LiquidOut) -> TankModel/2(LiquidOut)
  Memory/1 -> Control/8(LiquidLevel)
  MR3/1 -> Control/3(ManualReference)
  CT3/1 -> Control/2(StartMaintenance), Control/1(ControlType)
  F3/1 -> Control/4(Fill)
  E3/1 -> Control/5(Empty)
  EB3/1 -> Control/6(EmergencyButton)
  T3/1 -> Control/7(Temperature)
  Control/1(LiquidIn) -> TankModel/1(LiquidIn)

== system c00004M_harness/M222/Tank3 ==
  CT3 : Inport
  F3 : Inport  Port=2
  E3 : Inport  Port=3
  MR3 : Inport  Port=4
  T3 : Inport  Port=5
  EB3 : Inport  Port=6
  Control : Subsystem
  Memory : Memory
  TankModel : Subsystem
  LL3 : Outport
  wires:
  TankModel/1(LiquidLevel) -> Memory/1, LL3/1
  Control/2(LiquidOut) -> TankModel/2(LiquidOut)
  Memory/1 -> Control/8(LiquidLevel)
  MR3/1 -> Control/3(ManualReference)
  CT3/1 -> Control/2(StartMaintenance), Control/1(ControlType)
  F3/1 -> Control/4(Fill)
  E3/1 -> Control/5(Empty)
  EB3/1 -> Control/6(EmergencyButton)
  T3/1 -> Control/7(Temperature)
  Control/1(LiquidIn) -> TankModel/1(LiquidIn)

== system c00004M_harness/M223/Tank3 ==
  CT3 : Inport
  F3 : Inport  Port=2
  E3 : Inport  Port=3
  MR3 : Inport  Port=4
  T3 : Inport  Port=5
  EB3 : Inport  Port=6
  Control : Subsystem
  Memory : Memory
  TankModel : Subsystem
  LL3 : Outport
  wires:
  TankModel/1(LiquidLevel) -> Memory/1, LL3/1
  Control/2(LiquidOut) -> TankModel/2(LiquidOut)
  Memory/1 -> Control/8(LiquidLevel)
  MR3/1 -> Control/3(ManualReference)
  CT3/1 -> Control/2(StartMaintenance), Control/1(ControlType)
  F3/1 -> Control/4(Fill)
  E3/1 -> Control/5(Empty)
  EB3/1 -> Control/6(EmergencyButton)
  T3/1 -> Control/7(Temperature)
  Control/1(LiquidIn) -> TankModel/1(LiquidIn)

== system c00004M_harness/M224/Tank3 ==
  CT3 : Inport
  F3 : Inport  Port=2
  E3 : Inport  Port=3
  MR3 : Inport  Port=4
  T3 : Inport  Port=5
  EB3 : Inport  Port=6
  Control : Subsystem
  Memory : Memory
  TankModel : Subsystem
  LL3 : Outport
  wires:
  TankModel/1(LiquidLevel) -> Memory/1, LL3/1
  Control/2(LiquidOut) -> TankModel/2(LiquidOut)
  Memory/1 -> Control/8(LiquidLevel)
  MR3/1 -> Control/3(ManualReference)
  CT3/1 -> Control/2(StartMaintenance), Control/1(ControlType)
  F3/1 -> Control/4(Fill)
  E3/1 -> Control/5(Empty)
  EB3/1 -> Control/6(EmergencyButton)
  T3/1 -> Control/7(Temperature)
  Control/1(LiquidIn) -> TankModel/1(LiquidIn)

== system c00004M_harness/M225/Tank3 ==
  CT3 : Inport
  F3 : Inport  Port=2
  E3 : Inport  Port=3
  MR3 : Inport  Port=4
  T3 : Inport  Port=5
  EB3 : Inport  Port=6
  Control : Subsystem
  Memory : Memory
  TankModel : Subsystem
  LL3 : Outport
  wires:
  TankModel/1(LiquidLevel) -> Memory/1, LL3/1
  Control/2(LiquidOut) -> TankModel/2(LiquidOut)
  Memory/1 -> Control/8(LiquidLevel)
  MR3/1 -> Control/3(ManualReference)
  CT3/1 -> Control/2(StartMaintenance), Control/1(ControlType)
  F3/1 -> Control/4(Fill)
  E3/1 -> Control/5(Empty)
  EB3/1 -> Control/6(EmergencyButton)
  T3/1 -> Control/7(Temperature)
  Control/1(LiquidIn) -> TankModel/1(LiquidIn)

== system c00004M_harness/M233/Tank3 ==
  CT3 : Inport
  F3 : Inport  Port=2
  E3 : Inport  Port=3
  MR3 : Inport  Port=4
  T3 : Inport  Port=5
  EB3 : Inport  Port=6
  Control : Subsystem
  Memory : Memory
  TankModel : Subsystem
  LL3 : Outport
  wires:
  TankModel/1(LiquidLevel) -> Memory/1, LL3/1
  Control/2(LiquidOut) -> TankModel/2(LiquidOut)
  Memory/1 -> Control/8(LiquidLevel)
  MR3/1 -> Control/3(ManualReference)
  CT3/1 -> Control/2(StartMaintenance), Control/1(ControlType)
  F3/1 -> Control/4(Fill)
  E3/1 -> Control/5(Empty)
  EB3/1 -> Control/6(EmergencyButton)
  T3/1 -> Control/7(Temperature)
  Control/1(LiquidIn) -> TankModel/1(LiquidIn)

== system c00004M_harness/M234/Tank3 ==
  CT3 : Inport
  F3 : Inport  Port=2
  E3 : Inport  Port=3
  MR3 : Inport  Port=4
  T3 : Inport  Port=5
  EB3 : Inport  Port=6
  Control : Subsystem
  Memory : Memory
  TankModel : Subsystem
  LL3 : Outport
  wires:
  TankModel/1(LiquidLevel) -> Memory/1, LL3/1
  Control/2(LiquidOut) -> TankModel/2(LiquidOut)
  Memory/1 -> Control/8(LiquidLevel)
  MR3/1 -> Control/3(ManualReference)
  CT3/1 -> Control/2(StartMaintenance), Control/1(ControlType)
  F3/1 -> Control/4(Fill)
  E3/1 -> Control/5(Empty)
  EB3/1 -> Control/6(EmergencyButton)
  T3/1 -> Control/7(Temperature)
  Control/1(LiquidIn) -> TankModel/1(LiquidIn)

== system c00004M_harness/M235/Tank3 ==
  CT3 : Inport
  F3 : Inport  Port=2
  E3 : Inport  Port=3
  MR3 : Inport  Port=4
  T3 : Inport  Port=5
  EB3 : Inport  Port=6
  Control : Subsystem
  Memory : Memory
  TankModel : Subsystem
  LL3 : Outport
  wires:
  TankModel/1(LiquidLevel) -> Memory/1, LL3/1
  Control/2(LiquidOut) -> TankModel/2(LiquidOut)
  Memory/1 -> Control/8(LiquidLevel)
  MR3/1 -> Control/3(ManualReference)
  CT3/1 -> Control/2(StartMaintenance), Control/1(ControlType)
  F3/1 -> Control/4(Fill)
  E3/1 -> Control/5(Empty)
  EB3/1 -> Control/6(EmergencyButton)
  T3/1 -> Control/7(Temperature)
  Control/1(LiquidIn) -> TankModel/1(LiquidIn)

== system c00004M_harness/M236/Tank3 ==
  CT3 : Inport
  F3 : Inport  Port=2
  E3 : Inport  Port=3
  MR3 : Inport  Port=4
  T3 : Inport  Port=5
  EB3 : Inport  Port=6
  Control : Subsystem
  Memory : Memory
  TankModel : Subsystem
  LL3 : Outport
  wires:
  TankModel/1(LiquidLevel) -> Memory/1, LL3/1
  Control/2(LiquidOut) -> TankModel/2(LiquidOut)
  Memory/1 -> Control/8(LiquidLevel)
  MR3/1 -> Control/3(ManualReference)
  CT3/1 -> Control/2(StartMaintenance), Control/1(ControlType)
  F3/1 -> Control/4(Fill)
  E3/1 -> Control/5(Empty)
  EB3/1 -> Control/6(EmergencyButton)
  T3/1 -> Control/7(Temperature)
  Control/1(LiquidIn) -> TankModel/1(LiquidIn)

== system c00004M_harness/M237/Tank3 ==
  CT3 : Inport
  F3 : Inport  Port=2
  E3 : Inport  Port=3
  MR3 : Inport  Port=4
  T3 : Inport  Port=5
  EB3 : Inport  Port=6
  Control : Subsystem
  Memory : Memory
  TankModel : Subsystem
  LL3 : Outport
  wires:
  TankModel/1(LiquidLevel) -> Memory/1, LL3/1
  Control/2(LiquidOut) -> TankModel/2(LiquidOut)
  Memory/1 -> Control/8(LiquidLevel)
  MR3/1 -> Control/3(ManualReference)
  CT3/1 -> Control/2(StartMaintenance), Control/1(ControlType)
  F3/1 -> Control/4(Fill)
  E3/1 -> Control/5(Empty)
  EB3/1 -> Control/6(EmergencyButton)
  T3/1 -> Control/7(Temperature)
  Control/1(LiquidIn) -> TankModel/1(LiquidIn)

== system c00004M_harness/M238/Tank3 ==
  CT3 : Inport
  F3 : Inport  Port=2
  E3 : Inport  Port=3
  MR3 : Inport  Port=4
  T3 : Inport  Port=5
  EB3 : Inport  Port=6
  Control : Subsystem
  Memory : Memory
  TankModel : Subsystem
  LL3 : Outport
  wires:
  TankModel/1(LiquidLevel) -> Memory/1, LL3/1
  Control/2(LiquidOut) -> TankModel/2(LiquidOut)
  Memory/1 -> Control/8(LiquidLevel)
  MR3/1 -> Control/3(ManualReference)
  CT3/1 -> Control/2(StartMaintenance), Control/1(ControlType)
  F3/1 -> Control/4(Fill)
  E3/1 -> Control/5(Empty)
  EB3/1 -> Control/6(EmergencyButton)
  T3/1 -> Control/7(Temperature)
  Control/1(LiquidIn) -> TankModel/1(LiquidIn)

== system c00004M_harness/M239/Tank3 ==
  CT3 : Inport
  F3 : Inport  Port=2
  E3 : Inport  Port=3
  MR3 : Inport  Port=4
  T3 : Inport  Port=5
  EB3 : Inport  Port=6
  Control : Subsystem
  Memory : Memory
  TankModel : Subsystem
  LL3 : Outport
  wires:
  TankModel/1(LiquidLevel) -> Memory/1, LL3/1
  Control/2(LiquidOut) -> TankModel/2(LiquidOut)
  Memory/1 -> Control/8(LiquidLevel)
  MR3/1 -> Control/3(ManualReference)
  CT3/1 -> Control/2(StartMaintenance), Control/1(ControlType)
  F3/1 -> Control/4(Fill)
  E3/1 -> Control/5(Empty)
  EB3/1 -> Control/6(EmergencyButton)
  T3/1 -> Control/7(Temperature)
  Control/1(LiquidIn) -> TankModel/1(LiquidIn)

== system c00004M_harness/M240/Tank3 ==
  CT3 : Inport
  F3 : Inport  Port=2
  E3 : Inport  Port=3
  MR3 : Inport  Port=4
  T3 : Inport  Port=5
  EB3 : Inport  Port=6
  Control : Subsystem
  Memory : Memory
  TankModel : Subsystem
  LL3 : Outport
  wires:
  TankModel/1(LiquidLevel) -> Memory/1, LL3/1
  Control/2(LiquidOut) -> TankModel/2(LiquidOut)
  Memory/1 -> Control/8(LiquidLevel)
  MR3/1 -> Control/3(ManualReference)
  CT3/1 -> Control/2(StartMaintenance), Control/1(ControlType)
  F3/1 -> Control/4(Fill)
  E3/1 -> Control/5(Empty)
  EB3/1 -> Control/6(EmergencyButton)
  T3/1 -> Control/7(Temperature)
  Control/1(LiquidIn) -> TankModel/1(LiquidIn)

== system c00004M_harness/M241/Tank3 ==
  CT3 : Inport
  F3 : Inport  Port=2
  E3 : Inport  Port=3
  MR3 : Inport  Port=4
  T3 : Inport  Port=5
  EB3 : Inport  Port=6
  Control : Subsystem
  Memory : Memory
  TankModel : Subsystem
  LL3 : Outport
  wires:
  TankModel/1(LiquidLevel) -> Memory/1, LL3/1
  Control/2(LiquidOut) -> TankModel/2(LiquidOut)
  Memory/1 -> Control/8(LiquidLevel)
  MR3/1 -> Control/3(ManualReference)
  CT3/1 -> Control/2(StartMaintenance), Control/1(ControlType)
  F3/1 -> Control/4(Fill)
  E3/1 -> Control/5(Empty)
  EB3/1 -> Control/6(EmergencyButton)
  T3/1 -> Control/7(Temperature)
  Control/1(LiquidIn) -> TankModel/1(LiquidIn)

== system c00004M_harness/M242/Tank3 ==
  CT3 : Inport
  F3 : Inport  Port=2
  E3 : Inport  Port=3
  MR3 : Inport  Port=4
  T3 : Inport  Port=5
  EB3 : Inport  Port=6
  Control : Subsystem
  Memory : Memory
  TankModel : Subsystem
  LL3 : Outport
  wires:
  TankModel/1(LiquidLevel) -> Memory/1, LL3/1
  Control/2(LiquidOut) -> TankModel/2(LiquidOut)
  Memory/1 -> Control/8(LiquidLevel)
  MR3/1 -> Control/3(ManualReference)
  CT3/1 -> Control/2(StartMaintenance), Control/1(ControlType)
  F3/1 -> Control/4(Fill)
  E3/1 -> Control/5(Empty)
  EB3/1 -> Control/6(EmergencyButton)
  T3/1 -> Control/7(Temperature)
  Control/1(LiquidIn) -> TankModel/1(LiquidIn)

== system c00004M_harness/M243/Tank3 ==
  CT3 : Inport
  F3 : Inport  Port=2
  E3 : Inport  Port=3
  MR3 : Inport  Port=4
  T3 : Inport  Port=5
  EB3 : Inport  Port=6
  Control : Subsystem
  Memory : Memory
  TankModel : Subsystem
  LL3 : Outport
  wires:
  TankModel/1(LiquidLevel) -> Memory/1, LL3/1
  Control/2(LiquidOut) -> TankModel/2(LiquidOut)
  Memory/1 -> Control/8(LiquidLevel)
  MR3/1 -> Control/3(ManualReference)
  CT3/1 -> Control/2(StartMaintenance), Control/1(ControlType)
  F3/1 -> Control/4(Fill)
  E3/1 -> Control/5(Empty)
  EB3/1 -> Control/6(EmergencyButton)
  T3/1 -> Control/7(Temperature)
  Control/1(LiquidIn) -> TankModel/1(LiquidIn)

== system c00004M_harness/M244/Tank3 ==
  CT3 : Inport
  F3 : Inport  Port=2
  E3 : Inport  Port=3
  MR3 : Inport  Port=4
  T3 : Inport  Port=5
  EB3 : Inport  Port=6
  Control : Subsystem
  Memory : Memory
  TankModel : Subsystem
  LL3 : Outport
  wires:
  TankModel/1(LiquidLevel) -> Memory/1, LL3/1
  Control/2(LiquidOut) -> TankModel/2(LiquidOut)
  Memory/1 -> Control/8(LiquidLevel)
  MR3/1 -> Control/3(ManualReference)
  CT3/1 -> Control/2(StartMaintenance), Control/1(ControlType)
  F3/1 -> Control/4(Fill)
  E3/1 -> Control/5(Empty)
  EB3/1 -> Control/6(EmergencyButton)
  T3/1 -> Control/7(Temperature)
  Control/1(LiquidIn) -> TankModel/1(LiquidIn)

== system c00004M_harness/M245/Tank3 ==
  CT3 : Inport
  F3 : Inport  Port=2
  E3 : Inport  Port=3
  MR3 : Inport  Port=4
  T3 : Inport  Port=5
  EB3 : Inport  Port=6
  Control : Subsystem
  Memory : Memory
  TankModel : Subsystem
  LL3 : Outport
  wires:
  TankModel/1(LiquidLevel) -> Memory/1, LL3/1
  Control/2(LiquidOut) -> TankModel/2(LiquidOut)
  Memory/1 -> Control/8(LiquidLevel)
  MR3/1 -> Control/3(ManualReference)
  CT3/1 -> Control/2(StartMaintenance), Control/1(ControlType)
  F3/1 -> Control/4(Fill)
  E3/1 -> Control/5(Empty)
  EB3/1 -> Control/6(EmergencyButton)
  T3/1 -> Control/7(Temperature)
  Control/1(LiquidIn) -> TankModel/1(LiquidIn)

== system c00004M_harness/M246/Tank3 ==
  CT3 : Inport
  F3 : Inport  Port=2
  E3 : Inport  Port=3
  MR3 : Inport  Port=4
  T3 : Inport  Port=5
  EB3 : Inport  Port=6
  Control : Subsystem
  Memory : Memory
  TankModel : Subsystem
  LL3 : Outport
  wires:
  TankModel/1(LiquidLevel) -> Memory/1, LL3/1
  Control/2(LiquidOut) -> TankModel/2(LiquidOut)
  Memory/1 -> Control/8(LiquidLevel)
  MR3/1 -> Control/3(ManualReference)
  CT3/1 -> Control/2(StartMaintenance), Control/1(ControlType)
  F3/1 -> Control/4(Fill)
  E3/1 -> Control/5(Empty)
  EB3/1 -> Control/6(EmergencyButton)
  T3/1 -> Control/7(Temperature)
  Control/1(LiquidIn) -> TankModel/1(LiquidIn)

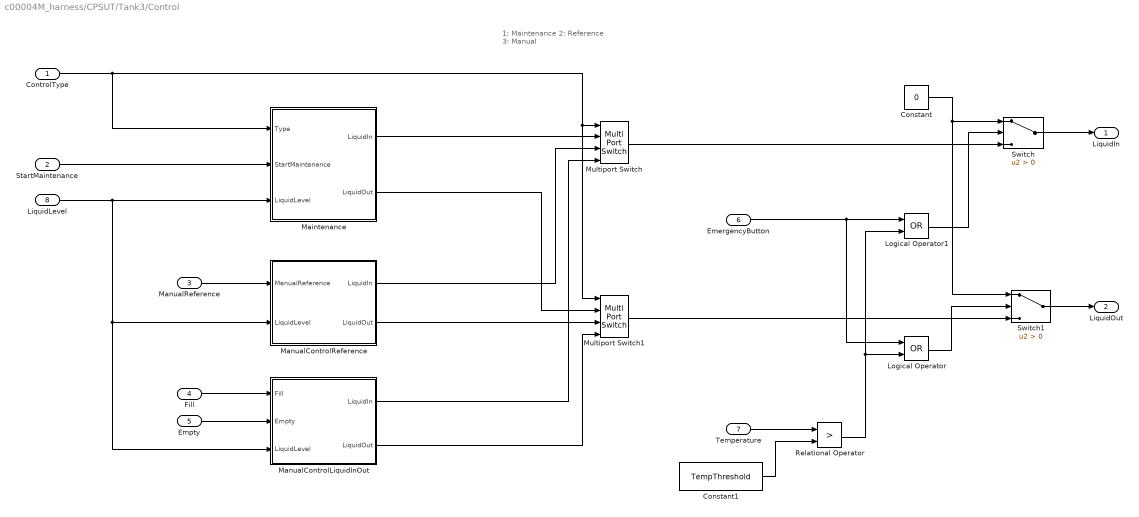
== system c00004M_harness/CPSUT/Tank3/Control ==
  note: 1: Maintenance
      | 2: Reference
      | 3: Manual
  ControlType : Inport
  StartMaintenance : Inport  Port=2
  ManualReference : Inport  Port=3
  Fill : Inport  Port=4
  Empty : Inport  Port=5
  EmergencyButton : Inport  Port=6
  Temperature : Inport  Port=7
  LiquidLevel : Inport  Port=8
  Constant : Constant  Value=0
  Constant1 : Constant  Value=TempThreshold
  Logical Operator : Logic  Operator=OR  AllPortsSameDT=off  OutDataTypeStr=boolean
  Logical Operator1 : Logic  Operator=OR  AllPortsSameDT=off  OutDataTypeStr=boolean
  Maintenance : Subsystem
  ManualControlLiquidInOut : Subsystem
  ManualControlReference : Subsystem
  Multiport Switch : MultiPortSwitch
  Multiport Switch1 : MultiPortSwitch
  Relational Operator : RelationalOperator  Operator=>  OutDataTypeStr=boolean  RndMeth=Simplest
  Switch : Switch  Criteria=u2 > Threshold
  Switch1 : Switch  Criteria=u2 > Threshold
  LiquidIn : Outport
  LiquidOut : Outport  Port=2
  wires:
  Multiport Switch/1 -> Switch/3
  Multiport Switch1/1 -> Switch1/3
  ControlType/1 -> Multiport Switch1/1, Multiport Switch/1, Maintenance/1(Type)
  Maintenance/1(LiquidIn) -> Multiport Switch/2
  ManualControlReference/1(LiquidIn) -> Multiport Switch/3
  Maintenance/2(LiquidOut) -> Multiport Switch1/2
  ManualControlReference/2(LiquidOut) -> Multiport Switch1/3
  ManualReference/1 -> ManualControlReference/1(ManualReference)
  LiquidLevel/1 -> ManualControlLiquidInOut/3(LiquidLevel), ManualControlReference/2(LiquidLevel), Maintenance/3(LiquidLevel)
  ManualControlLiquidInOut/1(LiquidIn) -> Multiport Switch/4
  ManualControlLiquidInOut/2(LiquidOut) -> Multiport Switch1/4
  Empty/1 -> ManualControlLiquidInOut/2(Empty)
  Fill/1 -> ManualControlLiquidInOut/1(Fill)
  StartMaintenance/1 -> Maintenance/2(StartMaintenance)
  Switch/1 -> LiquidIn/1
  Switch1/1 -> LiquidOut/1
  Constant/1 -> Switch1/1, Switch/1
  EmergencyButton/1 -> Logical Operator/1, Logical Operator1/1
  Relational Operator/1 -> Logical Operator1/2, Logical Operator/2
  Logical Operator/1 -> Switch1/2
  Logical Operator1/1 -> Switch/2
  Temperature/1 -> Relational Operator/1
  Constant1/1 -> Relational Operator/2

== system c00004M_harness/CPSUT/Tank3/TankModel ==
  LiquidIn : Inport
  LiquidOut : Inport  Port=2
  Add1 : Sum  Inputs=+-
  Constant1 : Constant  Value=0
  Constant2 : Constant  Value=0
  Constant3 : Constant
  Gain : Gain  Gain=1/R1
  Gain1 : Gain  Gain=1/A1
  Gain2 : Gain  Gain=1/R2
  Integrator : Integrator
  Saturation : Saturate  UpperLimit=hmax  LowerLimit=0
  Switch : Switch  Criteria=u2 ~= 0
  Switch1 : Switch  Criteria=u2 ~= 0
  LiquidLevel : Outport
  wires:
  Saturation/1 -> LiquidLevel/1, Gain2/1
  LiquidOut/1 -> Switch/2
  Add1/1 -> Gain1/1
  Gain2/1 -> Switch/1
  LiquidIn/1 -> Switch1/2
  Switch/1 -> Add1/2
  Switch1/1 -> Gain/1
  Constant2/1 -> Switch/3
  Constant3/1 -> Switch1/1
  Integrator/1 -> Saturation/1
  Gain1/1 -> Integrator/1
  Gain/1 -> Add1/1
  Constant1/1 -> Switch1/3

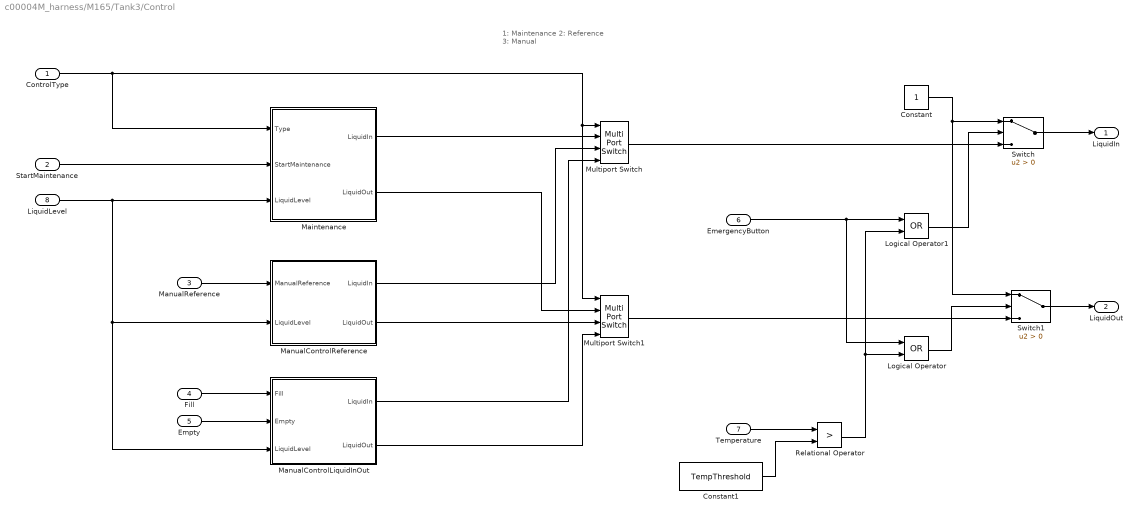
== system c00004M_harness/M165/Tank3/Control ==
  note: 1: Maintenance
      | 2: Reference
      | 3: Manual
  ControlType : Inport
  StartMaintenance : Inport  Port=2
  ManualReference : Inport  Port=3
  Fill : Inport  Port=4
  Empty : Inport  Port=5
  EmergencyButton : Inport  Port=6
  Temperature : Inport  Port=7
  LiquidLevel : Inport  Port=8
  Constant : Constant
  Constant1 : Constant  Value=TempThreshold
  Logical Operator : Logic  Operator=OR  AllPortsSameDT=off  OutDataTypeStr=boolean
  Logical Operator1 : Logic  Operator=OR  AllPortsSameDT=off  OutDataTypeStr=boolean
  Maintenance : Subsystem
  ManualControlLiquidInOut : Subsystem
  ManualControlReference : Subsystem
  Multiport Switch : MultiPortSwitch
  Multiport Switch1 : MultiPortSwitch
  Relational Operator : RelationalOperator  Operator=>  OutDataTypeStr=boolean  RndMeth=Simplest
  Switch : Switch  Criteria=u2 > Threshold
  Switch1 : Switch  Criteria=u2 > Threshold
  LiquidIn : Outport
  LiquidOut : Outport  Port=2
  wires:
  Multiport Switch/1 -> Switch/3
  Multiport Switch1/1 -> Switch1/3
  ControlType/1 -> Multiport Switch1/1, Multiport Switch/1, Maintenance/1(Type)
  Maintenance/1(LiquidIn) -> Multiport Switch/2
  ManualControlReference/1(LiquidIn) -> Multiport Switch/3
  Maintenance/2(LiquidOut) -> Multiport Switch1/2
  ManualControlReference/2(LiquidOut) -> Multiport Switch1/3
  ManualReference/1 -> ManualControlReference/1(ManualReference)
  LiquidLevel/1 -> ManualControlLiquidInOut/3(LiquidLevel), ManualControlReference/2(LiquidLevel), Maintenance/3(LiquidLevel)
  ManualControlLiquidInOut/1(LiquidIn) -> Multiport Switch/4
  ManualControlLiquidInOut/2(LiquidOut) -> Multiport Switch1/4
  Empty/1 -> ManualControlLiquidInOut/2(Empty)
  Fill/1 -> ManualControlLiquidInOut/1(Fill)
  StartMaintenance/1 -> Maintenance/2(StartMaintenance)
  Switch/1 -> LiquidIn/1
  Switch1/1 -> LiquidOut/1
  Constant/1 -> Switch1/1, Switch/1
  EmergencyButton/1 -> Logical Operator/1, Logical Operator1/1
  Relational Operator/1 -> Logical Operator1/2, Logical Operator/2
  Logical Operator/1 -> Switch1/2
  Logical Operator1/1 -> Switch/2
  Temperature/1 -> Relational Operator/1
  Constant1/1 -> Relational Operator/2

== system c00004M_harness/M165/Tank3/TankModel ==
  LiquidIn : Inport
  LiquidOut : Inport  Port=2
  Add1 : Sum  Inputs=+-
  Constant1 : Constant  Value=0
  Constant2 : Constant  Value=0
  Constant3 : Constant
  Gain : Gain  Gain=1/R1
  Gain1 : Gain  Gain=1/A1
  Gain2 : Gain  Gain=1/R2
  Integrator : Integrator
  Saturation : Saturate  UpperLimit=hmax  LowerLimit=0
  Switch : Switch  Criteria=u2 ~= 0
  Switch1 : Switch  Criteria=u2 ~= 0
  LiquidLevel : Outport
  wires:
  Saturation/1 -> LiquidLevel/1, Gain2/1
  LiquidOut/1 -> Switch/2
  Add1/1 -> Gain1/1
  Gain2/1 -> Switch/1
  LiquidIn/1 -> Switch1/2
  Switch/1 -> Add1/2
  Switch1/1 -> Gain/1
  Constant2/1 -> Switch/3
  Constant3/1 -> Switch1/1
  Integrator/1 -> Saturation/1
  Gain1/1 -> Integrator/1
  Gain/1 -> Add1/1
  Constant1/1 -> Switch1/3
